simulink model "gm_ZynqBF_2tx_fpga"  (R2018b)
settings: Solver=FixedStepDiscrete  StartTime=0.0  StopTime=10.0  RelTol=1e-3
settings Model: Creator=jason  LastModifiedBy=jason
settings DataIOCC: SaveOutput=off  SaveTime=off
settings OptimizationCC: BlockReduction=off  ConditionallyExecuteInputs=off  DefaultParameterBehavior=Inlined
settings DebuggingCC: AlgebraicLoopMsg=error  InheritedTsInSrcMsg=none  SingleTaskRateTransMsg=error  StrictBusMsg=ErrorOnBusTreatedAsVector
settings HardwareCC: ProdBitPerPointer=32  ProdBitPerSizeT=32  ProdBitPerPtrDiffT=32  ProdLargestAtomicFloat=None  ProdIntDivRoundTo=Undefined  ProdEndianess=Unspecified  ProdWordSize=32  ProdHWDeviceType=ASIC/FPGA->ASIC/FPGA  ProdEqTarget=off
settings SFSimCC: SimUseLocalCustomCode=off
settings RTWCC: RTWUseLocalCustomCode=off
settings CodeAppCC: StateflowObjectComments=on
settings GRTTargetCC: TargetLangStandard=C89/C90 (ANSI)

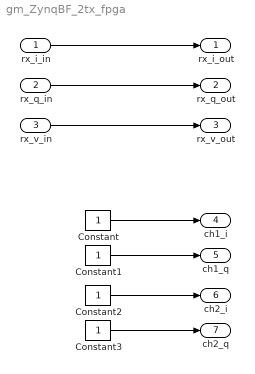
== system gm_ZynqBF_2tx_fpga ==
  rx_i_in : Inport  OutDataTypeStr=fixdt(1, 16, 15)  PortDimensions=1  SampleTime=0.2
  rx_q_in : Inport  Port=2  OutDataTypeStr=fixdt(1, 16, 15)  PortDimensions=1  SampleTime=0.2
  rx_v_in : Inport  Port=3  OutDataTypeStr=boolean  PortDimensions=1  SampleTime=0.2
  Constant{,1..3} (4 alike) : Constant  OutDataTypeStr=fixdt(1,16,15)  SampleTime=-1
  rx_i_out : Outport  OutDataTypeStr=fixdt(1,16,15)
  rx_q_out : Outport  Port=2  OutDataTypeStr=fixdt(1,16,15)
  rx_v_out : Outport  Port=3  OutDataTypeStr=boolean  LockScale=on
  ch1_i : Outport  Port=4  OutDataTypeStr=fixdt(1,16,15)
  ch1_q : Outport  Port=5  OutDataTypeStr=fixdt(1,16,15)
  ch2_i : Outport  Port=6  OutDataTypeStr=fixdt(1,16,15)
  ch2_q : Outport  Port=7  OutDataTypeStr=fixdt(1,16,15)
  wires:
  rx_i_in/1 -> rx_i_out/1
  rx_q_in/1 -> rx_q_out/1
  rx_v_in/1 -> rx_v_out/1
  Constant/1 -> ch1_i/1
  Constant1/1 -> ch1_q/1
  Constant2/1 -> ch2_i/1
  Constant3/1 -> ch2_q/1
